simulink model "Kalman_PhaseAndEM_Simple"  (R2019b)
settings: Solver=VariableStepAuto  StartTime=0.0  StopTime=model.sim_dur  FixedStep=model.Ts  RelTol=1e-6
undefined symbols (not defined in the file or in its folder): a_curr, f_curr, model, sigmaR_curr
libraries: dspsrcs4 x7, dspindex x6
settings Model: Creator=isidoraradenkovic  LastModifiedBy=isidoraradenkovic

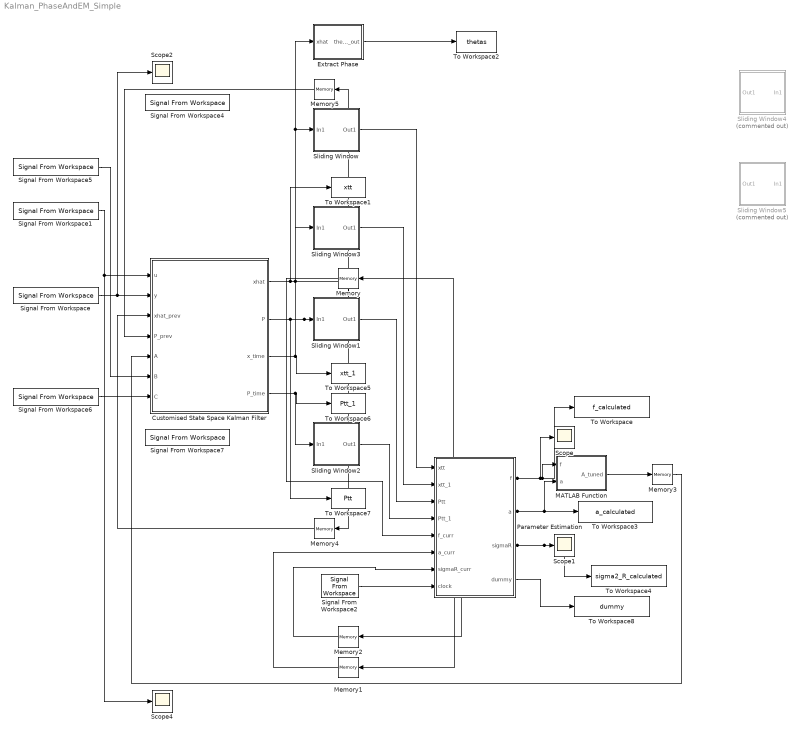
== system Kalman_PhaseAndEM_Simple ==
  Customised State Space Kalman Filter : MATLAB Function  TreatAsAtomicUnit=on
  Extract Phase : MATLAB Function  TreatAsAtomicUnit=on  SystemSampleTime=model.Ts
  MATLAB Function : MATLAB Function  TreatAsAtomicUnit=on  SystemSampleTime=model.Ts
  Memory : Memory  InitialCondition=f_curr  InheritSampleTime=on
  Memory1 : Memory  InitialCondition=a_curr  InheritSampleTime=on
  Memory2 : Memory  InitialCondition=sigmaR_curr  InheritSampleTime=on
  Memory3 : Memory  InitialCondition=model.A  InheritSampleTime=on
  Memory4 : Memory  InitialCondition=model.x_0  InheritSampleTime=on
  Memory5 : Memory  InitialCondition=model.Q  InheritSampleTime=on
  Parameter Estimation : MATLAB Function  TreatAsAtomicUnit=on  SystemSampleTime=model.Ts
  Scope{,1..2,4} (4 alike) : Scope
  Signal From Workspace : dspsrcs4/Signal From Workspace  X=input_data  Ts=model.Ts  nsamps=1  OutputAfterFinalValue=Cyclic repetition  ignoreOrWarnInputAndFrameLengths=off  OutputFrames=off
  Signal From Workspace1 : dspsrcs4/Signal From Workspace  X=tms_pulses  Ts=model.Ts  nsamps=1  OutputAfterFinalValue=Cyclic repetition  ignoreOrWarnInputAndFrameLengths=off  OutputFrames=off
  Signal From Workspace2 : dspsrcs4/Signal From Workspace  X=1:1:(6*model.param_est_length)  Ts=model.Ts  nsamps=1  OutputAfterFinalValue=Holding final value  ignoreOrWarnInputAndFrameLengths=off  OutputFrames=off
  Signal From Workspace4 : dspsrcs4/Signal From Workspace  X=model.A  Ts=model.Ts/2  nsamps=2  OutputAfterFinalValue=Cyclic repetition  ignoreOrWarnInputAndFrameLengths=off  OutputFrames=off
  Signal From Workspace5 : dspsrcs4/Signal From Workspace  X=model.B  Ts=model.Ts/2  nsamps=2  OutputAfterFinalValue=Cyclic repetition  ignoreOrWarnInputAndFrameLengths=off  OutputFrames=off
  Signal From Workspace6 : dspsrcs4/Signal From Workspace  X=model.C  Ts=model.Ts  nsamps=1  OutputAfterFinalValue=Cyclic repetition  ignoreOrWarnInputAndFrameLengths=off  OutputFrames=off
  Signal From Workspace7 : dspsrcs4/Signal From Workspace  X=model.D  Ts=model.Ts  nsamps=1  OutputAfterFinalValue=Cyclic repetition  ignoreOrWarnInputAndFrameLengths=off  OutputFrames=off
  Sliding Window : Subsystem
  Sliding Window1 : Subsystem
  Sliding Window2 : Subsystem
  Sliding Window3 : Subsystem
  Sliding Window4 : Subsystem  Commented=on
  Sliding Window5 : Subsystem  Commented=on
  To Workspace : ToWorkspace  VariableName=f_calculated  SampleTime=model.Ts
      settings: MaxDataPoints=1  Save2DSignal=2-D array (concatenate along first dimension)
  To Workspace1 : ToWorkspace  VariableName=xtt  SampleTime=model.Ts
      settings: Save2DSignal=2-D array (concatenate along first dimension)
  To Workspace2 : ToWorkspace  VariableName=thetas  SampleTime=model.Ts
      settings: Save2DSignal=2-D array (concatenate along first dimension)
  To Workspace3 : ToWorkspace  VariableName=a_calculated  SampleTime=model.Ts
      settings: MaxDataPoints=2  Save2DSignal=2-D array (concatenate along first dimension)
  To Workspace4 : ToWorkspace  VariableName=sigma2_R_calculated  SampleTime=model.Ts
      settings: MaxDataPoints=1  Save2DSignal=2-D array (concatenate along first dimension)
  To Workspace5 : ToWorkspace  VariableName=xtt_1  SampleTime=model.Ts
      settings: Save2DSignal=2-D array (concatenate along first dimension)
  To Workspace6 : ToWorkspace  VariableName=Ptt_1  SampleTime=model.Ts
      settings: Save2DSignal=2-D array (concatenate along first dimension)
  To Workspace7 : ToWorkspace  VariableName=Ptt  SampleTime=model.Ts
      settings: Save2DSignal=2-D array (concatenate along first dimension)
  To Workspace8 : ToWorkspace  VariableName=dummy  SampleTime=model.Ts
      settings: Save2DSignal=2-D array (concatenate along first dimension)
  wires:
  Signal From Workspace/1 -> Scope2/1, Customised State Space Kalman Filter/2(y)
  Signal From Workspace1/1 -> Scope4/1, Customised State Space Kalman Filter/1(u)
  Parameter Estimation/3(sigmaR) -> To Workspace4/1, Scope1/1, Memory2/1
  Parameter Estimation/2(a) -> MATLAB Function/2(a), To Workspace3/1, Memory1/1
  Memory2/1 -> Parameter Estimation/7(sigmaR_curr)
  Parameter Estimation/1(f) -> MATLAB Function/1(f), To Workspace/1, Scope/1, Memory/1
  Customised State Space Kalman Filter/4(P_time) -> To Workspace6/1, Sliding Window2/1(In1)
  Customised State Space Kalman Filter/3(x_time) -> Sliding Window3/1(In1), To Workspace5/1
  Customised State Space Kalman Filter/2(P) -> Sliding Window1/1(In1), Memory5/1, To Workspace7/1
  Signal From Workspace2/1 -> Parameter Estimation/8(clock)
  Sliding Window3/1(Out1) -> Parameter Estimation/2(xtt_1)
  MATLAB Function/1(A_tuned) -> Memory3/1
  Signal From Workspace6/1 -> Customised State Space Kalman Filter/7(C)
  Memory4/1 -> Customised State Space Kalman Filter/3(xhat_prev)
  Sliding Window1/1(Out1) -> Parameter Estimation/3(Ptt)
  Sliding Window2/1(Out1) -> Parameter Estimation/4(Ptt_1)
  Parameter Estimation/4(dummy) -> To Workspace8/1
  Memory3/1 -> Customised State Space Kalman Filter/5(A)
  Customised State Space Kalman Filter/1(xhat) -> Sliding Window/1(In1), Extract Phase/1(xhat), Memory4/1, To Workspace1/1
  Sliding Window/1(Out1) -> Parameter Estimation/1(xtt)
  Memory5/1 -> Customised State Space Kalman Filter/4(P_prev)
  Memory1/1 -> Parameter Estimation/6(a_curr)
  Extract Phase/1(thetas_out) -> To Workspace2/1
  Signal From Workspace5/1 -> Customised State Space Kalman Filter/6(B)
  Memory/1 -> Parameter Estimation/5(f_curr)

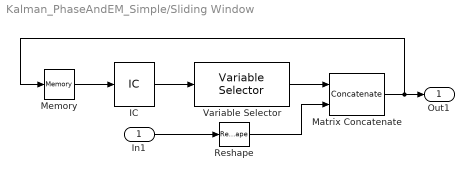
== system Kalman_PhaseAndEM_Simple/Sliding Window ==
  In1 : Inport
  IC : InitialCondition  Value=zeros(model.param_est_length+1, 2)
  Matrix Concatenate : Concatenate  Mode=Multidimensional array
  Memory : Memory  InheritSampleTime=on
  Reshape : Reshape  OutputDimensionality=Row vector (2-D)
  Variable Selector : dspindex/Variable Selector  NumInputs=1  rowsOrCols=Rows  IdxMode=Fixed  Elements=2:(model.param_est_length+1)  ZerOneIdxMode=One-based  errmode=Clip Index  FillMode=on  FillValues=0
  Out1 : Outport
  wires:
  Matrix Concatenate/1 -> Memory/1, Out1/1
  IC/1 -> Variable Selector/1
  Memory/1 -> IC/1
  In1/1 -> Reshape/1
  Variable Selector/1 -> Matrix Concatenate/1
  Reshape/1 -> Matrix Concatenate/2

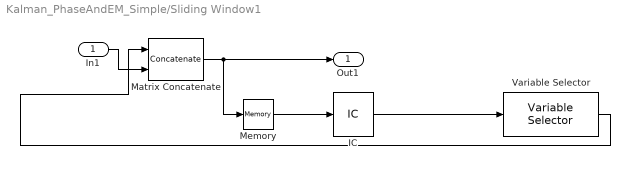
== system Kalman_PhaseAndEM_Simple/Sliding Window1 ==
  In1 : Inport
  IC : InitialCondition  Value=zeros(2*(model.param_est_length+1), 2)
  Matrix Concatenate : Concatenate  Mode=Multidimensional array
  Memory : Memory  InheritSampleTime=on
  Variable Selector : dspindex/Variable Selector  NumInputs=1  rowsOrCols=Rows  IdxMode=Fixed  Elements=3:2*(model.param_est_length+1)  ZerOneIdxMode=One-based  errmode=Clip Index  FillMode=on  FillValues=0
  Out1 : Outport
  wires:
  Matrix Concatenate/1 -> Out1/1, Memory/1
  IC/1 -> Variable Selector/1
  Variable Selector/1 -> Matrix Concatenate/1
  Memory/1 -> IC/1
  In1/1 -> Matrix Concatenate/2

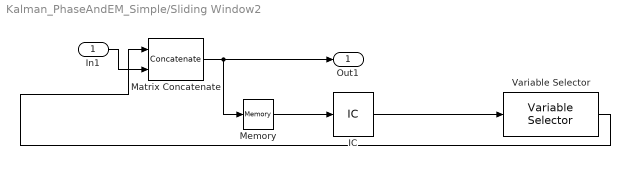
== system Kalman_PhaseAndEM_Simple/Sliding Window2 ==
  In1 : Inport
  IC : InitialCondition  Value=zeros(2*(model.param_est_length+1), 2)
  Matrix Concatenate : Concatenate  Mode=Multidimensional array
  Memory : Memory  InheritSampleTime=on
  Variable Selector : dspindex/Variable Selector  NumInputs=1  rowsOrCols=Rows  IdxMode=Fixed  Elements=3:2*(model.param_est_length+1)  ZerOneIdxMode=One-based  errmode=Clip Index  FillMode=on  FillValues=0
  Out1 : Outport
  wires:
  Matrix Concatenate/1 -> Out1/1, Memory/1
  IC/1 -> Variable Selector/1
  Variable Selector/1 -> Matrix Concatenate/1
  Memory/1 -> IC/1
  In1/1 -> Matrix Concatenate/2

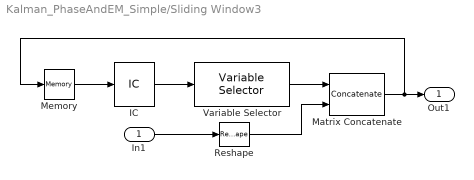
== system Kalman_PhaseAndEM_Simple/Sliding Window3 ==
  In1 : Inport
  IC : InitialCondition  Value=zeros(model.param_est_length+1, 2)
  Matrix Concatenate : Concatenate  Mode=Multidimensional array
  Memory : Memory  InheritSampleTime=on
  Reshape : Reshape  OutputDimensionality=Row vector (2-D)
  Variable Selector : dspindex/Variable Selector  NumInputs=1  rowsOrCols=Rows  IdxMode=Fixed  Elements=2:(model.param_est_length+1)  ZerOneIdxMode=One-based  errmode=Clip Index  FillMode=on  FillValues=0
  Out1 : Outport
  wires:
  IC/1 -> Variable Selector/1
  Memory/1 -> IC/1
  Variable Selector/1 -> Matrix Concatenate/1
  In1/1 -> Reshape/1
  Matrix Concatenate/1 -> Out1/1, Memory/1
  Reshape/1 -> Matrix Concatenate/2

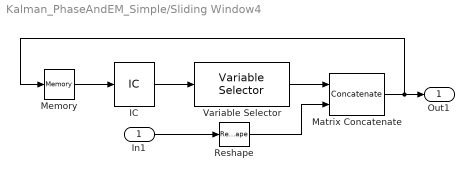
== system Kalman_PhaseAndEM_Simple/Sliding Window4 ==
  In1 : Inport
  IC : InitialCondition  Value=zeros(model.window, 2)
  Matrix Concatenate : Concatenate  Mode=Multidimensional array
  Memory : Memory  InheritSampleTime=on
  Reshape : Reshape  OutputDimensionality=Row vector (2-D)
  Variable Selector : dspindex/Variable Selector  NumInputs=1  rowsOrCols=Rows  IdxMode=Fixed  Elements=2:model.window  ZerOneIdxMode=One-based  errmode=Clip Index  FillMode=on  FillValues=0
  Out1 : Outport
  wires:
  Matrix Concatenate/1 -> Memory/1, Out1/1
  IC/1 -> Variable Selector/1
  Memory/1 -> IC/1
  In1/1 -> Reshape/1
  Variable Selector/1 -> Matrix Concatenate/1
  Reshape/1 -> Matrix Concatenate/2

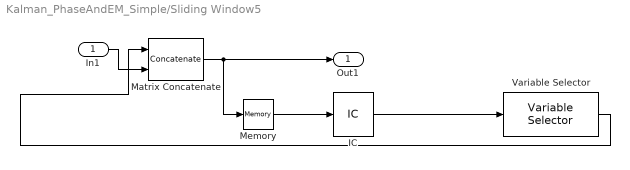
== system Kalman_PhaseAndEM_Simple/Sliding Window5 ==
  In1 : Inport
  IC : InitialCondition  Value=zeros(2*model.window, 2)
  Matrix Concatenate : Concatenate  Mode=Multidimensional array
  Memory : Memory  InheritSampleTime=on
  Variable Selector : dspindex/Variable Selector  NumInputs=1  rowsOrCols=Rows  IdxMode=Fixed  Elements=3:2*model.window  ZerOneIdxMode=One-based  errmode=Clip Index  FillMode=on  FillValues=0
  Out1 : Outport
  wires:
  Matrix Concatenate/1 -> Out1/1, Memory/1
  IC/1 -> Variable Selector/1
  Variable Selector/1 -> Matrix Concatenate/1
  Memory/1 -> IC/1
  In1/1 -> Matrix Concatenate/2

== matlab function Kalman_PhaseAndEM_Simple/Parameter Estimation ==
  settings: sampleTime=1
  data: xtt input; xtt_1 input; Ptt input; f output size=model.num_rhythms; Ptt_1 input; a output size=[2*model.num_rhythms, 2*model.num_rhythms]; sigmaR output size=model.num_rhythms; model parameter; f_curr input; a_curr input; sigmaR_curr input; clock input; dummy output
function [f, a, sigmaR, dummy]  = parameter_estimation(xtt, xtt_1, Ptt, Ptt_1, model, f_curr, a_curr, sigmaR_curr, clock)

%WARNING!!!!!! To-do: add dimensions_param = model.state_dimensions;
%Right now, 2 is used as a dimension because Simulink complains when
%variables are used for matrix dimensions. When the state space is
%extended for artefact removal, change the 2's to a new value.
%Warning No2: note the limits imposed on model parameters, such as how
%many samples we use to do EM. If this starts causing errors, ensure
%that you are using last n samples where n is at most the max used here.
%model = model;

if clock >= model.param_est_length+2 && clock <= model.param_est_length+5
    %%Backward Smoothing
    [PttN, xttN, Ptt_1N, xforwN, PforwN] = backward_smoothing(model, Ptt, Ptt_1, xtt, xtt_1);
    
    %%EM parameter estimation
    [f, a, sigmaR, dummy]  = em_method(model, PttN, xttN, Ptt_1N, xforwN, PforwN);
    
else
    f = f_curr;
    a = a_curr;
    sigmaR = sigmaR_curr;
    dummy = [1 2; 3 4];
end

    function [PttN, xttN, Ptt_1N, xNfinal, PNfinal] = backward_smoothing(model, Ptt, Ptt_1, xtt, xtt_1)
        length_param = model.param_est_length; %Limit to a max of 5000, BUT product limit is 10000
        
        PttN = zeros(min(2 * length_param, 10000), 2); % For the smoothing step
        xttN = zeros(min(length_param, 5000), 2);
        Ptt_1N = zeros(min(2 * length_param, 10000), 2); % Covariance
        
        xforwN = xtt(length_param+1, :);
        PforwN = Ptt((2 * length_param+1):(2 * (length_param+1)), :);
        
        xNfinal = xforwN;
        PNfinal = PforwN;
        
        for j= (length_param+1):(-1):2 % The paper is 0 indexed, MATLAB is 1 indexed
            % Extract matrices for simpler representation
            % Index (j-1) becomes:
            % ((j-2)*dimensions_param+1):((j-1)*dimensions_param)
            % Index j becomes:
            % ((j-1)*dimensions_param+1):(j*dimensions_param)
            
            ind_prev = max((j-2)*2+1, 1):min((j-1)*2, 50000);
            ind_curr = max((j-1)*2+1, 1):min(j*2, 50000);
            
            Pt_1_prev = Ptt_1(ind_prev, :);
            Pt_1_curr = Ptt_1(ind_curr, :);
            %Pt_prev = Ptt(ind_prev, :);
            xt_prev = xtt_1(j-1, 1:2);
            
            J = Pt_1_prev*model.A'*pinv(Pt_1_curr);
            xttN(j-1, min(1:2, 10:11)) = xt_prev+(xforwN-xt_prev*(model.A'))*(J');
            PttN(ind_prev, min(1:2, 10:11)) = Pt_1_prev+J*(PforwN-Pt_1_curr)*J';
            %covariance is symmetric, so Ptt_1N = Pt_1tN = J*PttN hence:
            Ptt_1N(ind_prev, min(1:2, 10:11)) = J*PforwN;
            
            xforwN = xttN(j-1, :);
            PforwN = PttN(ind_prev, :);
        end
        
    end

    function [f, a, sigmaR, dummy]  = em_method(model, PttN, xttN, Ptt_1N, xNfinal, PNfinal)
        length_param = model.param_est_length;
        num_rhythms = model.num_rhythms;
        
        P_A = matrix_sum(PttN, 2);
        P_B = matrix_sum(Ptt_1N, 2);
        P_C = matrix_sum([PttN((2+1):end, :); PNfinal], 2);
        
        xtN = [xttN(2:min(length_param, 5000), :); xNfinal];
        x_A_prod = matrix_product(xttN, xttN, 2);
        x_A = matrix_sum(x_A_prod, 2);
        x_B_prod = matrix_product(xtN, xttN, 2);
        x_B = matrix_sum(x_B_prod, 2);
        x_C_prod = matrix_product(xtN, xtN, 2);
        x_C = matrix_sum(x_C_prod, 2);
        
        A_smooth = P_A+x_A;
        B_smooth = P_B+x_B;
        C_smooth = P_C+x_C;
        
        denum_temp = tr(B_smooth, num_rhythms);
        denum = denum_temp(1);
        f_temp = 0.5*pi;
        if denum ~= 0
            f_temp = atan(double(rt(B_smooth, num_rhythms))./double(tr(B_smooth, num_rhythms)));
        end
        
        a_temp = sqrt(rt(B_smooth, num_rhythms).^2+tr(B_smooth, num_rhythms).^2)./tr(A_smooth, num_rhythms);
        sigmaR_temp = double(tr(C_smooth, num_rhythms)-(a_temp.^2).*tr(A_smooth, num_rhythms))./double(2*length_param);
        
        %f_temp2 = mod(double(f_temp(1)/pi+50000), 2)*pi;
        f = f_temp(1);
        %f = length(f_temp);
        a = a_temp(1)*eye(2);
        sigmaR = sigmaR_temp(1);
        dummy = P_A;
    end

end

== matlab function Kalman_PhaseAndEM_Simple/Extract Phase ==
  settings: updateMethod=DISCRETE  sampleTime=model.Ts
  data: xhat input; thetas_out output
function thetas_out  = extract_phase(xhat)
num_rhythms = length(xhat)/2;
% thetas_out = zeros(num_rhythms, 1);
% 
% for j = 1:num_rhythms
%     Im = xhat(2 * (j-1) + 2);
%     Re = xhat(2 * (j-1) + 1);
%     thetas_out(j, 1) = atan2(Im, Re);
% end

thetas_out = atan2(xhat(2:2:2*num_rhythms), xhat(1:2:2*(num_rhythms-1)+1))

== matlab function Kalman_PhaseAndEM_Simple/MATLAB Function ==
  data: A_tuned output; f input; a input; model parameter
function A_tuned = tune_A(f, a, model)
angles = 2*pi*model.Ts*f;
rot_cell = cell(1); % GENERALISE FOR MULTIPLE FREQ TRACKING

for j = 1:1 % model.num_rhythms GENERALISE FOR MULTIPLE FREQ TRACKING
    rot_j = [cos(angles(j)) -sin(angles(j)); sin(angles(j)) cos(angles(j))];
    rot_cell{j} = rot_j;
end
rot =blkdiag(rot_cell{1}); % GENERALISE FOR MULTIPLE FREQ TRACKING

A_tuned = a*rot;

== matlab function Kalman_PhaseAndEM_Simple/Customised State Space Kalman Filter ==
  data: u input; xhat output; y input; xhat_prev input; P_prev input; A input; B input; C input; P output; x_time output; P_time output; model parameter
function [xhat, P, x_time, P_time] = custom_state_space_kalman(u, y, xhat_prev, P_prev, A, B, C, model)
x_time = A*xhat_prev + B*u;
P_time = A*P_prev*A'+ model.Gm*model.Q*model.Gm';

K = P_time*(C')*pinv(C*P_time*C' + model.R);
epsilon = y - C*x_time;

xhat = x_time + K*epsilon;
P = P_time - K*C*P_time;
end
